simulink model "dspwavelet_fixpt"  (Simulink 8.3)
settings: Solver=FixedStepDiscrete  SolverMode=SingleTasking  StartTime=0.0  StopTime=1024  RelTol=1e-3
model workspace: external: MAT-File dspwlets.mat (data not in the file)
undefined symbols (not defined in the file or in its folder): lod, ts
undefined symbols (not defined in the file): hid, hir, lor
libraries: dspmlti4 x12, dspsigops x5, simulink x2, dspmisc x1, dspsrcs4 x1, dspstat3 x1
settings Model: Creator=The MathWorks Inc.  ExtModeTrigMode=oneshot  ExtModeArmWhenConnect=off
settings DataIOCC: LimitDataPoints=off  SaveOutput=off  SaveTime=off  SignalLoggingName=sigsOut
settings OptimizationCC: BlockReduction=off  BooleanDataType=off  ExpressionDepthLimit=2147483647  InitFltsAndDblsToZero=on  EfficientMapNaN2IntZero=off
settings DebuggingCC: SaveWithParameterizedLinksMsg=none  SignalResolutionControl=TryResolveAllWithWarning  SolverPrmCheckMsg=none  MultiTaskDSMMsg=warning  MultiTaskCondExecSysMsg=none  IntegerOverflowMsg=none  ParameterPrecisionLossMsg=none  FcnCallInpInsideContextMsg=UseLocalSettings  StrictBusMsg=None
settings HardwareCC: TargetUnknown=on
settings RTWCC: IncludeERTFirstTime=on
settings GRTTargetCC: TargetFcnLib=ansi_tfl_tmw.mat

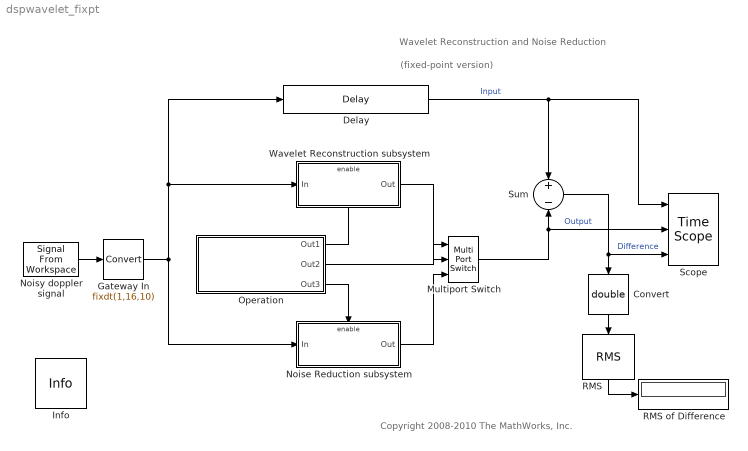
== system dspwavelet_fixpt ==
  note: Wavelet Reconstruction and Noise Reduction
  note: Copyright 2008-2010 The MathWorks, Inc.
  note: (fixed-point version)
  Convert : DataTypeConversion  OutDataTypeStr=double  RndMeth=Nearest  SaturateOnIntegerOverflow=on
  Delay : dspsigops/Delay  dly_unit=Samples  delay=7*(length(lod)-1)  ic_detail=on  dif_ic_for_ch=off  dif_ic_for_dly=off  ic=0  reset_popup=None
  Gateway In : DataTypeConversion  OutDataTypeStr=fixdt(1,16,10)  RndMeth=Nearest  SaturateOnIntegerOverflow=on
  Info : dspmisc/Info  SystemSampleTime=-1
  Multiport Switch : MultiPortSwitch  DataPortOrder=Zero-based contiguous  Inputs=2  zeroidx=on
  Noise Reduction subsystem : Subsystem  TreatAsAtomicUnit=on
  Noisy doppler signal : dspsrcs4/Signal From Workspace  X=noisdopp  Ts=ts  nsamps=1  OutputAfterFinalValue=Setting to zero  ignoreOrWarnInputAndFrameLengths=off
  Operation : Subsystem  mask(Wavelet Application){operation=Remove noise}
      mask help: Select a wavelet application
      mask init:
      | if operation == 1
      |     str = 'Perfect Reconstruction';
      | else
      |     str = 'Remove Noise';
      | end
      mask TypeOptions operation: Perfect reconstruction | Remove noise
      mask Display: disp(str)
  RMS : dspstat3/RMS  run=on  reset_popup=None  directionMode=Entire input  dimension=1  treatSBRowAsCol=on
  RMS of Difference : Display
  Scope : TimeScope  NumInputPorts=3  DefaultConfigurationName=spbscopes.TimeScopeBlockCfg  ScopeSpecification=DataTag10
  Sum : Sum  Inputs=+-  SaturateOnIntegerOverflow=on  InputSameDT=on  OutDataTypeStr=Inherit: Same as first input
  Wavelet Reconstruction subsystem : Subsystem  TreatAsAtomicUnit=on
  wires:
  Delay/1 -> Scope/1, Sum/1  "Input"
  Sum/1 -> Scope/3, Convert/1  "Difference"
  RMS/1 -> RMS of Difference/1
  Operation/1(Out1) -> Wavelet Reconstruction subsystem/Enable
  Wavelet Reconstruction subsystem/1(Out) -> Multiport Switch/2
  Noise Reduction subsystem/1(Out) -> Multiport Switch/3
  Noisy doppler signal/1 -> Gateway In/1
  Multiport Switch/1 -> Scope/2, Sum/2  "Output"
  Operation/2(Out2) -> Multiport Switch/1
  Operation/3(Out3) -> Noise Reduction subsystem/Enable
  Gateway In/1 -> Noise Reduction subsystem/1(In), Wavelet Reconstruction subsystem/1(In), Delay/1
  Convert/1 -> RMS/1

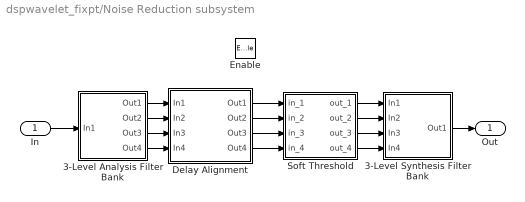
== system dspwavelet_fixpt/Noise Reduction subsystem ==
  In : Inport
  Enable : EnablePort
  3-Level Analysis Filter Bank : Subsystem
  3-Level Synthesis Filter Bank : Subsystem
  Delay Alignment : Subsystem
  Soft Threshold : Subsystem  mask(Soft Threshold){st=[3 2 1 0]}
      mask prompts: st "Vector of thresholds for each level:"
      mask help: Apply a soft threshold (deadzone transfer function) to each signal in the decomposition. First threshold applies to top-most filter bank output.
      mask init:
      | x=([-1 1 NaN 0 0 NaN -1 -.5 .5 1]+1)/2*.7+.15;
      | y=([0 0 NaN -1 1 NaN -1 0 0 1]+1)/2*.7+.05;
      mask Help: Vector of thresholds for each decomposition level.
      mask Display:
      | text(.1,.9,'Dead Zone')
      | plot(x,y)
  Out : Outport
  wires:
  Soft Threshold/1(out_1) -> 3-Level Synthesis Filter Bank/1(In1)
  Soft Threshold/2(out_2) -> 3-Level Synthesis Filter Bank/2(In2)
  Soft Threshold/3(out_3) -> 3-Level Synthesis Filter Bank/3(In3)
  Soft Threshold/4(out_4) -> 3-Level Synthesis Filter Bank/4(In4)
  3-Level Analysis Filter Bank/1(Out1) -> Delay Alignment/1(In1)
  3-Level Analysis Filter Bank/2(Out2) -> Delay Alignment/2(In2)
  3-Level Analysis Filter Bank/3(Out3) -> Delay Alignment/3(In3)
  3-Level Analysis Filter Bank/4(Out4) -> Delay Alignment/4(In4)
  Delay Alignment/1(Out1) -> Soft Threshold/1(in_1)
  Delay Alignment/2(Out2) -> Soft Threshold/2(in_2)
  Delay Alignment/3(Out3) -> Soft Threshold/3(in_3)
  Delay Alignment/4(Out4) -> Soft Threshold/4(in_4)
  In/1 -> 3-Level Analysis Filter Bank/1(In1)
  3-Level Synthesis Filter Bank/1(Out1) -> Out/1

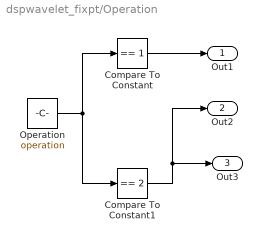
== system dspwavelet_fixpt/Operation ==
  Compare To Constant : simulink/Logic and Bit Operations/Compare To Constant  relop===  const=1  OutDataTypeStr=uint8  ZeroCross=off
  Compare To Constant1 : simulink/Logic and Bit Operations/Compare To Constant  relop===  const=2  OutDataTypeStr=uint8  ZeroCross=off
  Operation : Constant  Value=operation
  Out1 : Outport
  Out2 : Outport  Port=2
  Out3 : Outport  Port=3
  wires:
  Operation/1 -> Compare To Constant/1, Compare To Constant1/1
  Compare To Constant/1 -> Out1/1
  Compare To Constant1/1 -> Out3/1, Out2/1

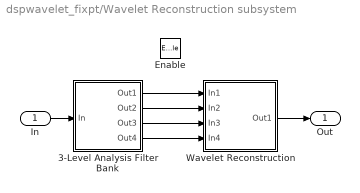
== system dspwavelet_fixpt/Wavelet Reconstruction subsystem ==
  In : Inport
  Enable : EnablePort
  3-Level Analysis Filter Bank : Subsystem  mask{low=lod, high=hid}
      mask prompts: low "Lowpass FIR filter coefficients:"; high "Highpass FIR filter coefficients:"
  Wavelet Reconstruction : Subsystem
  Out : Outport
  wires:
  In/1 -> 3-Level Analysis Filter Bank/1(In)
  3-Level Analysis Filter Bank/1(Out1) -> Wavelet Reconstruction/1(In1)
  3-Level Analysis Filter Bank/2(Out2) -> Wavelet Reconstruction/2(In2)
  3-Level Analysis Filter Bank/3(Out3) -> Wavelet Reconstruction/3(In3)
  3-Level Analysis Filter Bank/4(Out4) -> Wavelet Reconstruction/4(In4)
  Wavelet Reconstruction/1(Out1) -> Out/1

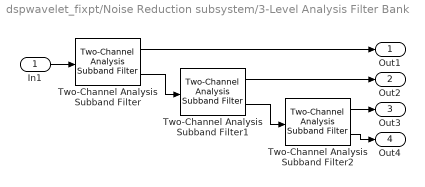
== system dspwavelet_fixpt/Noise Reduction subsystem/3-Level Analysis Filter Bank ==
  In1 : Inport
  Two-Channel Analysis Subband Filter : dspmlti4/Two-Channel Analysis Subband Filter  lpf=lod  hpf=hid  framing=Maintain input frame size  firstCoeffDataTypeStr=Inherit: Same word length as input  firstCoeffLastDataTypeStr=Inherit: Same word length as input  firstCoeffMin=[]  firstCoeffMax=[]  outputMin=[]  outputMax=[]  accumDataTypeStr=Inherit: Same as product output  accumLastDataTypeStr=Inherit: Same as product output  roundingMode=Floor  overflowMode=off
  Two-Channel Analysis Subband Filter1 : dspmlti4/Two-Channel Analysis Subband Filter  lpf=lod  hpf=hid  framing=Maintain input frame size  firstCoeffDataTypeStr=Inherit: Same word length as input  firstCoeffLastDataTypeStr=Inherit: Same word length as input  firstCoeffMin=[]  firstCoeffMax=[]  outputMin=[]  outputMax=[]  accumDataTypeStr=Inherit: Same as product output  accumLastDataTypeStr=Inherit: Same as product output  roundingMode=Floor  overflowMode=off
  Two-Channel Analysis Subband Filter2 : dspmlti4/Two-Channel Analysis Subband Filter  lpf=lod  hpf=hid  framing=Maintain input frame size  firstCoeffDataTypeStr=Inherit: Same word length as input  firstCoeffLastDataTypeStr=Inherit: Same word length as input  firstCoeffMin=[]  firstCoeffMax=[]  outputMin=[]  outputMax=[]  accumDataTypeStr=Inherit: Same as product output  accumLastDataTypeStr=Inherit: Same as product output  roundingMode=Floor  overflowMode=off
  Out1 : Outport
  Out2 : Outport  Port=2
  Out3 : Outport  Port=3
  Out4 : Outport  Port=4
  wires:
  Two-Channel Analysis Subband Filter2/2 -> Out4/1
  Two-Channel Analysis Subband Filter2/1 -> Out3/1
  Two-Channel Analysis Subband Filter1/1 -> Out2/1
  In1/1 -> Two-Channel Analysis Subband Filter/1
  Two-Channel Analysis Subband Filter/1 -> Out1/1
  Two-Channel Analysis Subband Filter1/2 -> Two-Channel Analysis Subband Filter2/1
  Two-Channel Analysis Subband Filter/2 -> Two-Channel Analysis Subband Filter1/1

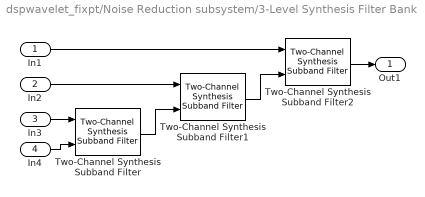
== system dspwavelet_fixpt/Noise Reduction subsystem/3-Level Synthesis Filter Bank ==
  In1 : Inport
  In2 : Inport  Port=2
  In3 : Inport  Port=3
  In4 : Inport  Port=4
  Two-Channel Synthesis Subband Filter : dspmlti4/Two-Channel Synthesis Subband Filter  lpf=lor  hpf=hir  framing=Maintain input frame size  firstCoeffDataTypeStr=Inherit: Same word length as input  firstCoeffLastDataTypeStr=Inherit: Same word length as input  firstCoeffMin=[]  firstCoeffMax=[]  outputDataTypeStr=Inherit: Same as accumulator  outputLastDataTypeStr=Inherit: Same as accumulator  outputMin=[]  outputMax=[]  accumDataTypeStr=Inherit: Same as product output  accumLastDataTypeStr=Inherit: Same as product output  roundingMode=Floor  overflowMode=off
  Two-Channel Synthesis Subband Filter1 : dspmlti4/Two-Channel Synthesis Subband Filter  lpf=lor  hpf=hir  framing=Maintain input frame size  firstCoeffDataTypeStr=Inherit: Same word length as input  firstCoeffLastDataTypeStr=Inherit: Same word length as input  firstCoeffMin=[]  firstCoeffMax=[]  outputDataTypeStr=Inherit: Same as accumulator  outputLastDataTypeStr=Inherit: Same as accumulator  outputMin=[]  outputMax=[]  accumDataTypeStr=Inherit: Same as product output  accumLastDataTypeStr=Inherit: Same as product output  roundingMode=Floor  overflowMode=off
  Two-Channel Synthesis Subband Filter2 : dspmlti4/Two-Channel Synthesis Subband Filter  lpf=lor  hpf=hir  framing=Maintain input frame size  firstCoeffDataTypeStr=Inherit: Same word length as input  firstCoeffLastDataTypeStr=Inherit: Same word length as input  firstCoeffMin=[]  firstCoeffMax=[]  outputDataTypeStr=Inherit: Same as accumulator  outputLastDataTypeStr=Inherit: Same as accumulator  outputMin=[]  outputMax=[]  accumDataTypeStr=Inherit: Same as product output  accumLastDataTypeStr=Inherit: Same as product output  roundingMode=Floor  overflowMode=off
  Out1 : Outport
  wires:
  In4/1 -> Two-Channel Synthesis Subband Filter/2
  In3/1 -> Two-Channel Synthesis Subband Filter/1
  In2/1 -> Two-Channel Synthesis Subband Filter1/1
  Two-Channel Synthesis Subband Filter2/1 -> Out1/1
  In1/1 -> Two-Channel Synthesis Subband Filter2/1
  Two-Channel Synthesis Subband Filter1/1 -> Two-Channel Synthesis Subband Filter2/2
  Two-Channel Synthesis Subband Filter/1 -> Two-Channel Synthesis Subband Filter1/2

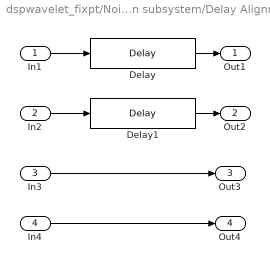
== system dspwavelet_fixpt/Noise Reduction subsystem/Delay Alignment ==
  In1 : Inport
  In2 : Inport  Port=2
  In3 : Inport  Port=3
  In4 : Inport  Port=4
  Delay : dspsigops/Delay  dly_unit=Samples  delay=3*(length(lod)-1)  ic_detail=on  dif_ic_for_ch=off  dif_ic_for_dly=off  ic=0  reset_popup=None
  Delay1 : dspsigops/Delay  dly_unit=Samples  delay=length(lod) - 1  ic_detail=on  dif_ic_for_ch=off  dif_ic_for_dly=off  ic=0  reset_popup=None
  Out1 : Outport
  Out2 : Outport  Port=2
  Out3 : Outport  Port=3
  Out4 : Outport  Port=4
  wires:
  In3/1 -> Out3/1
  In4/1 -> Out4/1
  In2/1 -> Delay1/1
  Delay1/1 -> Out2/1
  In1/1 -> Delay/1
  Delay/1 -> Out1/1

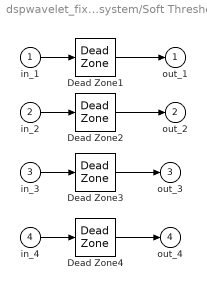
== system dspwavelet_fixpt/Noise Reduction subsystem/Soft Threshold ==
  in_1 : Inport
  in_2 : Inport  Port=2
  in_3 : Inport  Port=3
  in_4 : Inport  Port=4
  Dead Zone1 : DeadZone  LowerValue=-st(1)  UpperValue=st(1)  ZeroCross=off  SaturateOnIntegerOverflow=on
  Dead Zone2 : DeadZone  LowerValue=-st(2)  UpperValue=st(2)  ZeroCross=off  SaturateOnIntegerOverflow=on
  Dead Zone3 : DeadZone  LowerValue=-st(3)  UpperValue=st(3)  ZeroCross=off  SaturateOnIntegerOverflow=on
  Dead Zone4 : DeadZone  LowerValue=-st(4)  UpperValue=st(4)  ZeroCross=off  SaturateOnIntegerOverflow=on
  out_1 : Outport
  out_2 : Outport  Port=2
  out_3 : Outport  Port=3
  out_4 : Outport  Port=4
  wires:
  in_1/1 -> Dead Zone1/1
  Dead Zone1/1 -> out_1/1
  in_2/1 -> Dead Zone2/1
  Dead Zone2/1 -> out_2/1
  in_3/1 -> Dead Zone3/1
  Dead Zone3/1 -> out_3/1
  in_4/1 -> Dead Zone4/1
  Dead Zone4/1 -> out_4/1

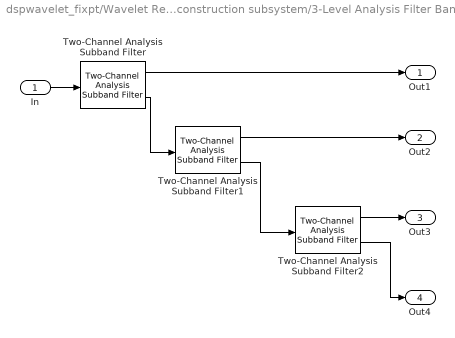
== system dspwavelet_fixpt/Wavelet Reconstruction subsystem/3-Level Analysis Filter Bank ==
  In : Inport
  Two-Channel Analysis Subband Filter : dspmlti4/Two-Channel Analysis Subband Filter  lpf=low  hpf=high  framing=Maintain input frame size  firstCoeffDataTypeStr=Inherit: Same word length as input  firstCoeffLastDataTypeStr=Inherit: Same word length as input  firstCoeffMin=[]  firstCoeffMax=[]  outputMin=[]  outputMax=[]  accumMode=Binary point scaling  accumWordLength=32  accumFracLength=25  accumDataTypeStr=fixdt(1,32,25)  accumLastDataTypeStr=fixdt(1,32,25)  roundingMode=Nearest  overflowMode=on
      settings: allowOverrides=off
  Two-Channel Analysis Subband Filter1 : dspmlti4/Two-Channel Analysis Subband Filter  lpf=low  hpf=high  framing=Maintain input frame size  firstCoeffDataTypeStr=Inherit: Same word length as input  firstCoeffLastDataTypeStr=Inherit: Same word length as input  firstCoeffMin=[]  firstCoeffMax=[]  outputMin=[]  outputMax=[]  accumMode=Binary point scaling  accumWordLength=32  accumFracLength=25  accumDataTypeStr=fixdt(1,32,25)  accumLastDataTypeStr=fixdt(1,32,25)  roundingMode=Nearest  overflowMode=on
      settings: allowOverrides=off
  Two-Channel Analysis Subband Filter2 : dspmlti4/Two-Channel Analysis Subband Filter  lpf=low  hpf=high  framing=Maintain input frame size  firstCoeffDataTypeStr=Inherit: Same word length as input  firstCoeffLastDataTypeStr=Inherit: Same word length as input  firstCoeffMin=[]  firstCoeffMax=[]  outputMin=[]  outputMax=[]  accumMode=Binary point scaling  accumWordLength=32  accumFracLength=25  accumDataTypeStr=fixdt(1,32,25)  accumLastDataTypeStr=fixdt(1,32,25)  roundingMode=Nearest  overflowMode=on
      settings: allowOverrides=off
  Out1 : Outport
  Out2 : Outport  Port=2
  Out3 : Outport  Port=3
  Out4 : Outport  Port=4
  wires:
  In/1 -> Two-Channel Analysis Subband Filter/1
  Two-Channel Analysis Subband Filter/1 -> Out1/1
  Two-Channel Analysis Subband Filter/2 -> Two-Channel Analysis Subband Filter1/1
  Two-Channel Analysis Subband Filter1/1 -> Out2/1
  Two-Channel Analysis Subband Filter2/1 -> Out3/1
  Two-Channel Analysis Subband Filter2/2 -> Out4/1
  Two-Channel Analysis Subband Filter1/2 -> Two-Channel Analysis Subband Filter2/1

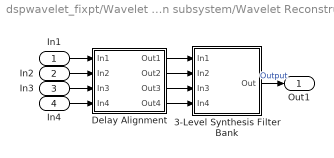
== system dspwavelet_fixpt/Wavelet Reconstruction subsystem/Wavelet Reconstruction ==
  In1 : Inport
  In2 : Inport  Port=2
  In3 : Inport  Port=3
  In4 : Inport  Port=4
  3-Level Synthesis Filter Bank : Subsystem  mask{low=lor, high=hir}
      mask prompts: low "Lowpass FIR filter coefficients:"; high "Highpass FIR filter coefficients:"
  Delay Alignment : Subsystem
  Out1 : Outport
  wires:
  In4/1 -> Delay Alignment/4(In4)
  In3/1 -> Delay Alignment/3(In3)
  3-Level Synthesis Filter Bank/1(Out) -> Out1/1  "Output"
  In2/1 -> Delay Alignment/2(In2)
  In1/1 -> Delay Alignment/1(In1)
  Delay Alignment/4(Out4) -> 3-Level Synthesis Filter Bank/4(In4)
  Delay Alignment/3(Out3) -> 3-Level Synthesis Filter Bank/3(In3)
  Delay Alignment/2(Out2) -> 3-Level Synthesis Filter Bank/2(In2)
  Delay Alignment/1(Out1) -> 3-Level Synthesis Filter Bank/1(In1)

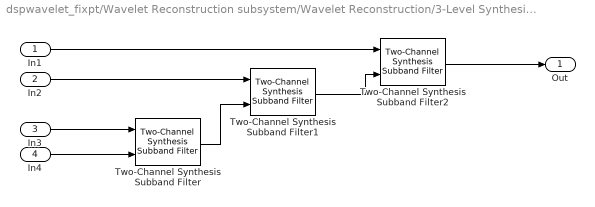
== system dspwavelet_fixpt/Wavelet Reconstruction subsystem/Wavelet Reconstruction/3-Level Synthesis Filter Bank ==
  In1 : Inport
  In2 : Inport  Port=2
  In3 : Inport  Port=3
  In4 : Inport  Port=4
  Two-Channel Synthesis Subband Filter : dspmlti4/Two-Channel Synthesis Subband Filter  lpf=low  hpf=high  framing=Maintain input frame size  firstCoeffDataTypeStr=Inherit: Same word length as input  firstCoeffLastDataTypeStr=Inherit: Same word length as input  firstCoeffMin=[]  firstCoeffMax=[]  outputMin=[]  outputMax=[]  accumMode=Binary point scaling  accumWordLength=32  accumFracLength=25  accumDataTypeStr=fixdt(1,32,25)  accumLastDataTypeStr=fixdt(1,32,25)  roundingMode=Nearest  overflowMode=on
      settings: allowOverrides=off
  Two-Channel Synthesis Subband Filter1 : dspmlti4/Two-Channel Synthesis Subband Filter  lpf=low  hpf=high  framing=Maintain input frame size  firstCoeffDataTypeStr=Inherit: Same word length as input  firstCoeffLastDataTypeStr=Inherit: Same word length as input  firstCoeffMin=[]  firstCoeffMax=[]  outputMin=[]  outputMax=[]  accumMode=Binary point scaling  accumWordLength=32  accumFracLength=25  accumDataTypeStr=fixdt(1,32,25)  accumLastDataTypeStr=fixdt(1,32,25)  roundingMode=Nearest  overflowMode=on
      settings: allowOverrides=off
  Two-Channel Synthesis Subband Filter2 : dspmlti4/Two-Channel Synthesis Subband Filter  lpf=low  hpf=high  framing=Maintain input frame size  firstCoeffDataTypeStr=Inherit: Same word length as input  firstCoeffLastDataTypeStr=Inherit: Same word length as input  firstCoeffMin=[]  firstCoeffMax=[]  outputMin=[]  outputMax=[]  accumMode=Binary point scaling  accumWordLength=32  accumFracLength=25  accumDataTypeStr=fixdt(1,32,25)  accumLastDataTypeStr=fixdt(1,32,25)  roundingMode=Nearest  overflowMode=on
      settings: allowOverrides=off
  Out : Outport
  wires:
  In3/1 -> Two-Channel Synthesis Subband Filter/1
  In4/1 -> Two-Channel Synthesis Subband Filter/2
  In2/1 -> Two-Channel Synthesis Subband Filter1/1
  Two-Channel Synthesis Subband Filter/1 -> Two-Channel Synthesis Subband Filter1/2
  In1/1 -> Two-Channel Synthesis Subband Filter2/1
  Two-Channel Synthesis Subband Filter1/1 -> Two-Channel Synthesis Subband Filter2/2
  Two-Channel Synthesis Subband Filter2/1 -> Out/1

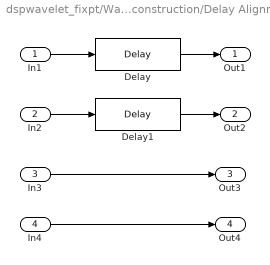
== system dspwavelet_fixpt/Wavelet Reconstruction subsystem/Wavelet Reconstruction/Delay Alignment ==
  In1 : Inport
  In2 : Inport  Port=2
  In3 : Inport  Port=3
  In4 : Inport  Port=4
  Delay : dspsigops/Delay  dly_unit=Samples  delay=3*(length(lod)-1)  ic_detail=off  dif_ic_for_ch=off  dif_ic_for_dly=off  ic=0  reset_popup=None
  Delay1 : dspsigops/Delay  dly_unit=Samples  delay=length(lod) - 1  ic_detail=off  dif_ic_for_ch=off  dif_ic_for_dly=off  ic=0  reset_popup=None
  Out1 : Outport
  Out2 : Outport  Port=2
  Out3 : Outport  Port=3
  Out4 : Outport  Port=4
  wires:
  Delay/1 -> Out1/1
  In1/1 -> Delay/1
  Delay1/1 -> Out2/1
  In2/1 -> Delay1/1
  In4/1 -> Out4/1
  In3/1 -> Out3/1
